simulink model "gm_uz_pmsm_model_6LUT_pd_vnl"  (R2023b)
settings: Solver=FixedStepAuto  StartTime=0.0  StopTime=0.05  RelTol=1e-3
PreLoadFcn:
  | uz_pmsm_model_init_parameter
PostLoadFcn:
  | % Import the data from Excel for a lookup table
  | FluxMapData = readtable('C:\Users\Philipp\ultrazohm\ultrazohm_sw\ip_cores\uz_pmsm_model\FluxMapData_2023-05-26_13-07-57.csv');
  | % Row indices for lookup table
  | d_current_in_d_axis = FluxMapData(8:27,1:end);
  | % Column indices for lookup table
  | q_current_in_d_axis = FluxMapData(29:48,1:end);
  | % Output values for lookup table
  | d_Flux_d_axis = FluxMapData(50:69,1:end);
undefined symbols (not defined in the file or in its folder): ad1, ad2, ad3, ad4, ad5, ad6, aq1, aq2, aq3, aq4, aq5, aq6, d_current_d_Flux, d_current_q_Flux, entkopplung_dynamic, entkopplung_linear, entkopplung_static, Fid1_Giq1, Fid2_Giq2, Flux_d, Flux_q, friction_coefficient, inertia, Ki_Bo_d, Ki_Bo_q, Kp_Bo_d, Kp_Bo_q, L_d, L_q, Ldq, parameter_nachfuerung, polepair, praediktion_entkopplung_nonlinear, psi_pm, q_current_d_Flux, q_current_q_Flux, R_1, simulate_mechanical, simulate_nonlinear_modell, simulate_open_loop, static_friction_torque, tau_sum, ts, ts_regler
libraries: hdlmdlgenlib x21, simulink x2, slpidlib x2
(part 3 of 4)

== system gm_uz_pmsm_model_6LUT_pd_vnl/uz_pmsm_model/Product110 ==
  In1 : Inport
  In2 : Inport  Port=2
  Product110 : Product  Inputs=**  OutDataTypeStr=single  SampleTime=1e-08
  Product110_pd1 : Delay  DelayLength=6
  Out1 : Outport
  wires:
  Product110_pd1/1 -> Out1/1
  Product110/1 -> Product110_pd1/1
  In2/1 -> Product110/2
  In1/1 -> Product110/1

== system gm_uz_pmsm_model_6LUT_pd_vnl/uz_pmsm_model/Product111 ==
  In1 : Inport
  In2 : Inport  Port=2
  Product111 : Product  Inputs=**  OutDataTypeStr=single  SampleTime=1e-08
  Product111_pd1 : Delay  DelayLength=6
  Out1 : Outport
  wires:
  Product111_pd1/1 -> Out1/1
  Product111/1 -> Product111_pd1/1
  In2/1 -> Product111/2
  In1/1 -> Product111/1

== system gm_uz_pmsm_model_6LUT_pd_vnl/uz_pmsm_model/Product12 ==
  In1 : Inport
  In2 : Inport  Port=2
  Product12 : Product  Inputs=**  OutDataTypeStr=single  SampleTime=1e-08
  Product12_pd1 : Delay  DelayLength=6
  Out1 : Outport
  wires:
  Product12_pd1/1 -> Out1/1
  Product12/1 -> Product12_pd1/1
  In2/1 -> Product12/2
  In1/1 -> Product12/1

== system gm_uz_pmsm_model_6LUT_pd_vnl/uz_pmsm_model/Product121 ==
  In1 : Inport
  In2 : Inport  Port=2
  Product121 : Product  Inputs=**  OutDataTypeStr=single  SampleTime=1e-08
  Product121_pd1 : Delay  DelayLength=6
  Out1 : Outport
  wires:
  Product121_pd1/1 -> Out1/1
  Product121/1 -> Product121_pd1/1
  In2/1 -> Product121/2
  In1/1 -> Product121/1

== system gm_uz_pmsm_model_6LUT_pd_vnl/uz_pmsm_model/Product122 ==
  In1 : Inport
  In2 : Inport  Port=2
  Product122 : Product  Inputs=**  OutDataTypeStr=single  SampleTime=1e-08
  Product122_pd1 : Delay  DelayLength=6
  Out1 : Outport
  wires:
  Product122_pd1/1 -> Out1/1
  Product122/1 -> Product122_pd1/1
  In2/1 -> Product122/2
  In1/1 -> Product122/1

== system gm_uz_pmsm_model_6LUT_pd_vnl/uz_pmsm_model/Product13 ==
  In1 : Inport
  In2 : Inport  Port=2
  Product13 : Product  Inputs=**  OutDataTypeStr=single  SampleTime=1e-08
  Product13_pd1 : Delay  DelayLength=6
  Out1 : Outport
  wires:
  Product13_pd1/1 -> Out1/1
  Product13/1 -> Product13_pd1/1
  In2/1 -> Product13/2
  In1/1 -> Product13/1

== system gm_uz_pmsm_model_6LUT_pd_vnl/uz_pmsm_model/Product131 ==
  In1 : Inport
  In2 : Inport  Port=2
  Product131 : Product  Inputs=**  OutDataTypeStr=single  SampleTime=1e-08
  Product131_pd1 : Delay  DelayLength=6
  Out1 : Outport
  wires:
  Product131_pd1/1 -> Out1/1
  Product131/1 -> Product131_pd1/1
  In2/1 -> Product131/2
  In1/1 -> Product131/1

== system gm_uz_pmsm_model_6LUT_pd_vnl/uz_pmsm_model/Product14 ==
  In1 : Inport
  In2 : Inport  Port=2
  Product14 : Product  Inputs=**  OutDataTypeStr=single  SampleTime=1e-08
  Product14_pd1 : Delay  DelayLength=6
  Out1 : Outport
  wires:
  Product14_pd1/1 -> Out1/1
  Product14/1 -> Product14_pd1/1
  In2/1 -> Product14/2
  In1/1 -> Product14/1

== system gm_uz_pmsm_model_6LUT_pd_vnl/uz_pmsm_model/Product141 ==
  In1 : Inport
  In2 : Inport  Port=2
  Product141 : Product  Inputs=**  OutDataTypeStr=single  SampleTime=1e-08
  Product141_pd1 : Delay  DelayLength=6
  Out1 : Outport
  wires:
  Product141_pd1/1 -> Out1/1
  Product141/1 -> Product141_pd1/1
  In2/1 -> Product141/2
  In1/1 -> Product141/1

== system gm_uz_pmsm_model_6LUT_pd_vnl/uz_pmsm_model/Product142 ==
  In1 : Inport
  In2 : Inport  Port=2
  Product142 : Product  Inputs=**  OutDataTypeStr=single  SampleTime=1e-08
  Product142_pd1 : Delay  DelayLength=6
  Out1 : Outport
  wires:
  Product142_pd1/1 -> Out1/1
  Product142/1 -> Product142_pd1/1
  In2/1 -> Product142/2
  In1/1 -> Product142/1

== system gm_uz_pmsm_model_6LUT_pd_vnl/uz_pmsm_model/Product15 ==
  In1 : Inport
  In2 : Inport  Port=2
  Product15 : Product  Inputs=**  OutDataTypeStr=single  SampleTime=1e-08
  Product15_pd1 : Delay  DelayLength=6
  Out1 : Outport
  wires:
  Product15_pd1/1 -> Out1/1
  Product15/1 -> Product15_pd1/1
  In2/1 -> Product15/2
  In1/1 -> Product15/1

== system gm_uz_pmsm_model_6LUT_pd_vnl/uz_pmsm_model/Product151 ==
  In1 : Inport
  In2 : Inport  Port=2
  Product151 : Product  Inputs=**  OutDataTypeStr=single  SampleTime=1e-08
  Product151_pd1 : Delay  DelayLength=6
  Out1 : Outport
  wires:
  Product151_pd1/1 -> Out1/1
  Product151/1 -> Product151_pd1/1
  In2/1 -> Product151/2
  In1/1 -> Product151/1

== system gm_uz_pmsm_model_6LUT_pd_vnl/uz_pmsm_model/Product16 ==
  In1 : Inport
  In2 : Inport  Port=2
  Product16 : Product  Inputs=**  OutDataTypeStr=single  SampleTime=1e-08
  Product16_pd1 : Delay  DelayLength=6
  Out1 : Outport
  wires:
  Product16_pd1/1 -> Out1/1
  Product16/1 -> Product16_pd1/1
  In2/1 -> Product16/2
  In1/1 -> Product16/1

== system gm_uz_pmsm_model_6LUT_pd_vnl/uz_pmsm_model/Product17 ==
  In1 : Inport
  In2 : Inport  Port=2
  Product17 : Product  Inputs=**  OutDataTypeStr=single  SampleTime=1e-08
  Product17_pd1 : Delay  DelayLength=6
  Out1 : Outport
  wires:
  Product17_pd1/1 -> Out1/1
  Product17/1 -> Product17_pd1/1
  In2/1 -> Product17/2
  In1/1 -> Product17/1

== system gm_uz_pmsm_model_6LUT_pd_vnl/uz_pmsm_model/Product18 ==
  In1 : Inport
  In2 : Inport  Port=2
  Product18 : Product  Inputs=**  OutDataTypeStr=single  SampleTime=1e-08
  Product18_pd1 : Delay  DelayLength=6
  Out1 : Outport
  wires:
  Product18_pd1/1 -> Out1/1
  Product18/1 -> Product18_pd1/1
  In2/1 -> Product18/2
  In1/1 -> Product18/1

== system gm_uz_pmsm_model_6LUT_pd_vnl/uz_pmsm_model/Product19 ==
  In1 : Inport
  In2 : Inport  Port=2
  Product19 : Product  Inputs=**  OutDataTypeStr=single  SampleTime=1e-08
  Product19_pd1 : Delay  DelayLength=6
  Out1 : Outport
  wires:
  Product19_pd1/1 -> Out1/1
  Product19/1 -> Product19_pd1/1
  In2/1 -> Product19/2
  In1/1 -> Product19/1

== system gm_uz_pmsm_model_6LUT_pd_vnl/uz_pmsm_model/Product2 ==
  In1 : Inport
  In2 : Inport  Port=2
  Product2 : Product  Inputs=**  OutDataTypeStr=single  SampleTime=1e-08
  Product2_pd1 : Delay  DelayLength=6
  Out1 : Outport
  wires:
  Product2_pd1/1 -> Out1/1
  Product2/1 -> Product2_pd1/1
  In2/1 -> Product2/2
  In1/1 -> Product2/1

== system gm_uz_pmsm_model_6LUT_pd_vnl/uz_pmsm_model/Product20 ==
  In1 : Inport
  In2 : Inport  Port=2
  Product20 : Product  Inputs=**  OutDataTypeStr=single  SampleTime=1e-08
  Product20_pd1 : Delay  DelayLength=6
  Out1 : Outport
  wires:
  Product20_pd1/1 -> Out1/1
  Product20/1 -> Product20_pd1/1
  In2/1 -> Product20/2
  In1/1 -> Product20/1

== system gm_uz_pmsm_model_6LUT_pd_vnl/uz_pmsm_model/Product201 ==
  In1 : Inport
  In2 : Inport  Port=2
  Product201 : Product  Inputs=**  OutDataTypeStr=single  SampleTime=1e-08
  Product201_pd1 : Delay  DelayLength=6
  Out1 : Outport
  wires:
  Product201_pd1/1 -> Out1/1
  Product201/1 -> Product201_pd1/1
  In2/1 -> Product201/2
  In1/1 -> Product201/1

== system gm_uz_pmsm_model_6LUT_pd_vnl/uz_pmsm_model/Product202 ==
  In1 : Inport
  In2 : Inport  Port=2
  Product202 : Product  Inputs=**  OutDataTypeStr=single  SampleTime=1e-08
  Product202_pd1 : Delay  DelayLength=6
  Out1 : Outport
  wires:
  Product202_pd1/1 -> Out1/1
  Product202/1 -> Product202_pd1/1
  In2/1 -> Product202/2
  In1/1 -> Product202/1

== system gm_uz_pmsm_model_6LUT_pd_vnl/uz_pmsm_model/Product203 ==
  In1 : Inport
  In2 : Inport  Port=2
  Product203 : Product  Inputs=**  OutDataTypeStr=single  SampleTime=1e-08
  Product203_pd1 : Delay  DelayLength=6
  Out1 : Outport
  wires:
  Product203_pd1/1 -> Out1/1
  Product203/1 -> Product203_pd1/1
  In2/1 -> Product203/2
  In1/1 -> Product203/1

== system gm_uz_pmsm_model_6LUT_pd_vnl/uz_pmsm_model/Product204 ==
  In1 : Inport
  In2 : Inport  Port=2
  Product204 : Product  Inputs=**  OutDataTypeStr=single  SampleTime=1e-08
  Product204_pd1 : Delay  DelayLength=6
  Out1 : Outport
  wires:
  Product204_pd1/1 -> Out1/1
  Product204/1 -> Product204_pd1/1
  In2/1 -> Product204/2
  In1/1 -> Product204/1

== system gm_uz_pmsm_model_6LUT_pd_vnl/uz_pmsm_model/Product205 ==
  In1 : Inport
  In2 : Inport  Port=2
  Product205 : Product  Inputs=**  OutDataTypeStr=single  SampleTime=1e-08
  Product205_pd1 : Delay  DelayLength=6
  Out1 : Outport
  wires:
  Product205_pd1/1 -> Out1/1
  Product205/1 -> Product205_pd1/1
  In2/1 -> Product205/2
  In1/1 -> Product205/1

== system gm_uz_pmsm_model_6LUT_pd_vnl/uz_pmsm_model/Product206 ==
  In1 : Inport
  In2 : Inport  Port=2
  Product206 : Product  Inputs=**  OutDataTypeStr=single  SampleTime=1e-08
  Product206_pd1 : Delay  DelayLength=6
  Out1 : Outport
  wires:
  Product206_pd1/1 -> Out1/1
  Product206/1 -> Product206_pd1/1
  In2/1 -> Product206/2
  In1/1 -> Product206/1

== system gm_uz_pmsm_model_6LUT_pd_vnl/uz_pmsm_model/Product207 ==
  In1 : Inport
  In2 : Inport  Port=2
  Product207 : Product  Inputs=**  OutDataTypeStr=single  SampleTime=1e-08
  Product207_pd1 : Delay  DelayLength=6
  Out1 : Outport
  wires:
  Product207_pd1/1 -> Out1/1
  Product207/1 -> Product207_pd1/1
  In2/1 -> Product207/2
  In1/1 -> Product207/1

== system gm_uz_pmsm_model_6LUT_pd_vnl/uz_pmsm_model/Product21 ==
  In1 : Inport
  In2 : Inport  Port=2
  Product21 : Product  Inputs=**  OutDataTypeStr=single  SampleTime=1e-08
  Product21_pd1 : Delay  DelayLength=6
  Out1 : Outport
  wires:
  Product21_pd1/1 -> Out1/1
  Product21/1 -> Product21_pd1/1
  In2/1 -> Product21/2
  In1/1 -> Product21/1

== system gm_uz_pmsm_model_6LUT_pd_vnl/uz_pmsm_model/Product22 ==
  In1 : Inport
  In2 : Inport  Port=2
  Product22 : Product  Inputs=**  OutDataTypeStr=single  SampleTime=1e-08
  Product22_pd1 : Delay  DelayLength=6
  Out1 : Outport
  wires:
  Product22_pd1/1 -> Out1/1
  Product22/1 -> Product22_pd1/1
  In2/1 -> Product22/2
  In1/1 -> Product22/1

== system gm_uz_pmsm_model_6LUT_pd_vnl/uz_pmsm_model/Product23 ==
  In1 : Inport
  In2 : Inport  Port=2
  Product23 : Product  Inputs=**  OutDataTypeStr=single  SampleTime=1e-08
  Product23_pd1 : Delay  DelayLength=6
  Out1 : Outport
  wires:
  Product23_pd1/1 -> Out1/1
  Product23/1 -> Product23_pd1/1
  In2/1 -> Product23/2
  In1/1 -> Product23/1

== system gm_uz_pmsm_model_6LUT_pd_vnl/uz_pmsm_model/Product24 ==
  In1 : Inport
  In2 : Inport  Port=2
  Product24 : Product  Inputs=**  OutDataTypeStr=single  SampleTime=1e-08
  Product24_pd1 : Delay  DelayLength=6
  Out1 : Outport
  wires:
  Product24_pd1/1 -> Out1/1
  Product24/1 -> Product24_pd1/1
  In2/1 -> Product24/2
  In1/1 -> Product24/1

== system gm_uz_pmsm_model_6LUT_pd_vnl/uz_pmsm_model/Product25 ==
  In1 : Inport
  In2 : Inport  Port=2
  Product25 : Product  Inputs=**  OutDataTypeStr=single  SampleTime=1e-08
  Product25_pd1 : Delay  DelayLength=6
  Out1 : Outport
  wires:
  Product25_pd1/1 -> Out1/1
  Product25/1 -> Product25_pd1/1
  In2/1 -> Product25/2
  In1/1 -> Product25/1

== system gm_uz_pmsm_model_6LUT_pd_vnl/uz_pmsm_model/Product3 ==
  In1 : Inport
  In2 : Inport  Port=2
  Product3 : Product  Inputs=**  OutDataTypeStr=single  SampleTime=1e-08
  Product3_pd1 : Delay  DelayLength=6
  Out1 : Outport
  wires:
  Product3_pd1/1 -> Out1/1
  Product3/1 -> Product3_pd1/1
  In2/1 -> Product3/2
  In1/1 -> Product3/1

== system gm_uz_pmsm_model_6LUT_pd_vnl/uz_pmsm_model/Product31 ==
  In1 : Inport
  In2 : Inport  Port=2
  Product31 : Product  Inputs=**  OutDataTypeStr=single  SampleTime=1e-08
  Product31_pd1 : Delay  DelayLength=6
  Out1 : Outport
  wires:
  Product31_pd1/1 -> Out1/1
  Product31/1 -> Product31_pd1/1
  In2/1 -> Product31/2
  In1/1 -> Product31/1

== system gm_uz_pmsm_model_6LUT_pd_vnl/uz_pmsm_model/Product32 ==
  In1 : Inport
  In2 : Inport  Port=2
  Product32 : Product  Inputs=**  OutDataTypeStr=single  SampleTime=1e-08
  Product32_pd1 : Delay  DelayLength=6
  Out1 : Outport
  wires:
  Product32_pd1/1 -> Out1/1
  Product32/1 -> Product32_pd1/1
  In2/1 -> Product32/2
  In1/1 -> Product32/1

== system gm_uz_pmsm_model_6LUT_pd_vnl/uz_pmsm_model/Product33 ==
  In1 : Inport
  In2 : Inport  Port=2
  Product33 : Product  Inputs=**  OutDataTypeStr=single  SampleTime=1e-08
  Product33_pd1 : Delay  DelayLength=6
  Out1 : Outport
  wires:
  Product33_pd1/1 -> Out1/1
  Product33/1 -> Product33_pd1/1
  In2/1 -> Product33/2
  In1/1 -> Product33/1

== system gm_uz_pmsm_model_6LUT_pd_vnl/uz_pmsm_model/Product34 ==
  In1 : Inport
  In2 : Inport  Port=2
  Product34 : Product  Inputs=**  OutDataTypeStr=single  SampleTime=1e-08
  Product34_pd1 : Delay  DelayLength=6
  Out1 : Outport
  wires:
  Product34_pd1/1 -> Out1/1
  Product34/1 -> Product34_pd1/1
  In2/1 -> Product34/2
  In1/1 -> Product34/1

== system gm_uz_pmsm_model_6LUT_pd_vnl/uz_pmsm_model/Product35 ==
  In1 : Inport
  In2 : Inport  Port=2
  Product35 : Product  Inputs=**  OutDataTypeStr=single  SampleTime=1e-08
  Product35_pd1 : Delay  DelayLength=6
  Out1 : Outport
  wires:
  Product35_pd1/1 -> Out1/1
  Product35/1 -> Product35_pd1/1
  In2/1 -> Product35/2
  In1/1 -> Product35/1

== system gm_uz_pmsm_model_6LUT_pd_vnl/uz_pmsm_model/Product4 ==
  In1 : Inport
  In2 : Inport  Port=2
  Product4 : Product  Inputs=**  OutDataTypeStr=single  SampleTime=1e-08
  Product4_pd1 : Delay  DelayLength=6
  Out1 : Outport
  wires:
  Product4_pd1/1 -> Out1/1
  Product4/1 -> Product4_pd1/1
  In2/1 -> Product4/2
  In1/1 -> Product4/1

== system gm_uz_pmsm_model_6LUT_pd_vnl/uz_pmsm_model/Product41 ==
  In1 : Inport
  In2 : Inport  Port=2
  Product41 : Product  Inputs=**  OutDataTypeStr=single  SampleTime=1e-08
  Product41_pd1 : Delay  DelayLength=6
  Out1 : Outport
  wires:
  Product41_pd1/1 -> Out1/1
  Product41/1 -> Product41_pd1/1
  In2/1 -> Product41/2
  In1/1 -> Product41/1

== system gm_uz_pmsm_model_6LUT_pd_vnl/uz_pmsm_model/Product42 ==
  In1 : Inport
  In2 : Inport  Port=2
  Product42 : Product  Inputs=**  OutDataTypeStr=single  SampleTime=1e-08
  Product42_pd1 : Delay  DelayLength=6
  Out1 : Outport
  wires:
  Product42_pd1/1 -> Out1/1
  Product42/1 -> Product42_pd1/1
  In2/1 -> Product42/2
  In1/1 -> Product42/1

== system gm_uz_pmsm_model_6LUT_pd_vnl/uz_pmsm_model/Product43 ==
  In1 : Inport
  In2 : Inport  Port=2
  Product43 : Product  Inputs=**  OutDataTypeStr=single  SampleTime=1e-08
  Product43_pd1 : Delay  DelayLength=6
  Out1 : Outport
  wires:
  Product43_pd1/1 -> Out1/1
  Product43/1 -> Product43_pd1/1
  In2/1 -> Product43/2
  In1/1 -> Product43/1

== system gm_uz_pmsm_model_6LUT_pd_vnl/uz_pmsm_model/Product5 ==
  In1 : Inport
  In2 : Inport  Port=2
  Product5 : Product  Inputs=**  OutDataTypeStr=single  SampleTime=1e-08
  Product5_pd1 : Delay  DelayLength=6
  Out1 : Outport
  wires:
  Product5_pd1/1 -> Out1/1
  Product5/1 -> Product5_pd1/1
  In2/1 -> Product5/2
  In1/1 -> Product5/1

== system gm_uz_pmsm_model_6LUT_pd_vnl/uz_pmsm_model/Product51 ==
  In1 : Inport
  In2 : Inport  Port=2
  Product51 : Product  Inputs=**  OutDataTypeStr=single  SampleTime=1e-08
  Product51_pd1 : Delay  DelayLength=6
  Out1 : Outport
  wires:
  Product51_pd1/1 -> Out1/1
  Product51/1 -> Product51_pd1/1
  In2/1 -> Product51/2
  In1/1 -> Product51/1

== system gm_uz_pmsm_model_6LUT_pd_vnl/uz_pmsm_model/Product52 ==
  In1 : Inport
  In2 : Inport  Port=2
  Product52 : Product  Inputs=**  OutDataTypeStr=single  SampleTime=1e-08
  Product52_pd1 : Delay  DelayLength=6
  Out1 : Outport
  wires:
  Product52_pd1/1 -> Out1/1
  Product52/1 -> Product52_pd1/1
  In2/1 -> Product52/2
  In1/1 -> Product52/1

== system gm_uz_pmsm_model_6LUT_pd_vnl/uz_pmsm_model/Product6 ==
  In1 : Inport
  In2 : Inport  Port=2
  Product6 : Product  Inputs=**  OutDataTypeStr=single  SampleTime=1e-08
  Product6_pd1 : Delay  DelayLength=6
  Out1 : Outport
  wires:
  Product6_pd1/1 -> Out1/1
  Product6/1 -> Product6_pd1/1
  In2/1 -> Product6/2
  In1/1 -> Product6/1

== system gm_uz_pmsm_model_6LUT_pd_vnl/uz_pmsm_model/Product61 ==
  In1 : Inport
  In2 : Inport  Port=2
  Product61 : Product  Inputs=**  OutDataTypeStr=single  SampleTime=1e-08
  Product61_pd1 : Delay  DelayLength=6
  Out1 : Outport
  wires:
  Product61_pd1/1 -> Out1/1
  Product61/1 -> Product61_pd1/1
  In2/1 -> Product61/2
  In1/1 -> Product61/1

== system gm_uz_pmsm_model_6LUT_pd_vnl/uz_pmsm_model/Product7 ==
  In1 : Inport
  In2 : Inport  Port=2
  Product7 : Product  Inputs=**  OutDataTypeStr=single  SampleTime=1e-08
  Product7_pd1 : Delay  DelayLength=6
  Out1 : Outport
  wires:
  Product7_pd1/1 -> Out1/1
  Product7/1 -> Product7_pd1/1
  In2/1 -> Product7/2
  In1/1 -> Product7/1

== system gm_uz_pmsm_model_6LUT_pd_vnl/uz_pmsm_model/Product71 ==
  In1 : Inport
  In2 : Inport  Port=2
  Product71 : Product  Inputs=**  OutDataTypeStr=single  SampleTime=1e-08
  Product71_pd1 : Delay  DelayLength=6
  Out1 : Outport
  wires:
  Product71_pd1/1 -> Out1/1
  Product71/1 -> Product71_pd1/1
  In2/1 -> Product71/2
  In1/1 -> Product71/1

== system gm_uz_pmsm_model_6LUT_pd_vnl/uz_pmsm_model/Product8 ==
  In1 : Inport
  In2 : Inport  Port=2
  Product8 : Product  Inputs=**  OutDataTypeStr=single  SampleTime=1e-08
  Product8_pd1 : Delay  DelayLength=6
  Out1 : Outport
  wires:
  Product8_pd1/1 -> Out1/1
  Product8/1 -> Product8_pd1/1
  In2/1 -> Product8/2
  In1/1 -> Product8/1

== system gm_uz_pmsm_model_6LUT_pd_vnl/uz_pmsm_model/Product9 ==
  In1 : Inport
  In2 : Inport  Port=2
  Product9 : Product  Inputs=**  OutDataTypeStr=single  SampleTime=1e-08
  Product9_pd1 : Delay  DelayLength=6
  Out1 : Outport
  wires:
  Product9_pd1/1 -> Out1/1
  Product9/1 -> Product9_pd1/1
  In2/1 -> Product9/2
  In1/1 -> Product9/1

== system gm_uz_pmsm_model_6LUT_pd_vnl/uz_pmsm_model/Product91 ==
  In1 : Inport
  In2 : Inport  Port=2
  Product91 : Product  Inputs=**  OutDataTypeStr=single  SampleTime=1e-08
  Product91_pd1 : Delay  DelayLength=6
  Out1 : Outport
  wires:
  Product91_pd1/1 -> Out1/1
  Product91/1 -> Product91_pd1/1
  In2/1 -> Product91/2
  In1/1 -> Product91/1

== system gm_uz_pmsm_model_6LUT_pd_vnl/uz_pmsm_model/Product92 ==
  In1 : Inport
  In2 : Inport  Port=2
  Product92 : Product  Inputs=**  OutDataTypeStr=single  SampleTime=1e-08
  Product92_pd1 : Delay  DelayLength=6
  Out1 : Outport
  wires:
  Product92_pd1/1 -> Out1/1
  Product92/1 -> Product92_pd1/1
  In2/1 -> Product92/2
  In1/1 -> Product92/1

== system gm_uz_pmsm_model_6LUT_pd_vnl/uz_pmsm_model/Reciprocal1_recip ==
  In1 : Inport
  Reciprocal1_recip : Math  Operator=reciprocal  SampleTime=1e-08
  Reciprocal1_recip_pd1 : Delay  DelayLength=16
  Out1 : Outport
  wires:
  Reciprocal1_recip_pd1/1 -> Out1/1
  Reciprocal1_recip/1 -> Reciprocal1_recip_pd1/1
  In1/1 -> Reciprocal1_recip/1

== system gm_uz_pmsm_model_6LUT_pd_vnl/uz_pmsm_model/Reciprocal1_recip1 ==
  In1 : Inport
  Reciprocal1_recip1 : Math  Operator=reciprocal  SampleTime=1e-08
  Reciprocal1_recip1_pd1 : Delay  DelayLength=16
  Out1 : Outport
  wires:
  Reciprocal1_recip1_pd1/1 -> Out1/1
  Reciprocal1_recip1/1 -> Reciprocal1_recip1_pd1/1
  In1/1 -> Reciprocal1_recip1/1

== system gm_uz_pmsm_model_6LUT_pd_vnl/uz_pmsm_model/Reciprocal_recip ==
  In1 : Inport
  Reciprocal_recip : Math  Operator=reciprocal  SampleTime=1e-08
  Reciprocal_recip_pd1 : Delay  DelayLength=16
  Out1 : Outport
  wires:
  Reciprocal_recip_pd1/1 -> Out1/1
  Reciprocal_recip/1 -> Reciprocal_recip_pd1/1
  In1/1 -> Reciprocal_recip/1

== system gm_uz_pmsm_model_6LUT_pd_vnl/uz_pmsm_model/Reciprocal_recip1 ==
  In1 : Inport
  Reciprocal_recip1 : Math  Operator=reciprocal  SampleTime=1e-08
  Reciprocal_recip1_pd1 : Delay  DelayLength=16
  Out1 : Outport
  wires:
  Reciprocal_recip1_pd1/1 -> Out1/1
  Reciprocal_recip1/1 -> Reciprocal_recip1_pd1/1
  In1/1 -> Reciprocal_recip1/1

== system gm_uz_pmsm_model_6LUT_pd_vnl/uz_pmsm_model/Sign1 ==
  In1 : Inport
  Sign1 : Signum  SampleTime=1e-08
  Out1 : Outport
  wires:
  Sign1/1 -> Out1/1
  In1/1 -> Sign1/1

== system gm_uz_pmsm_model_6LUT_pd_vnl/uz_pmsm_model/Sum ==
  In1 : Inport
  In2 : Inport  Port=2
  Sum : Sum  OutDataTypeStr=single  SampleTime=1e-08
  Sum_pd1 : Delay  DelayLength=6
  Out1 : Outport
  wires:
  Sum_pd1/1 -> Out1/1
  Sum/1 -> Sum_pd1/1
  In2/1 -> Sum/2
  In1/1 -> Sum/1

== system gm_uz_pmsm_model_6LUT_pd_vnl/uz_pmsm_model/Sum1 ==
  In1 : Inport
  In2 : Inport  Port=2
  Sum1 : Sum  Inputs=+-  OutDataTypeStr=single  SampleTime=1e-08
  Sum1_pd1 : Delay  DelayLength=6
  Out1 : Outport
  wires:
  Sum1_pd1/1 -> Out1/1
  Sum1/1 -> Sum1_pd1/1
  In2/1 -> Sum1/2
  In1/1 -> Sum1/1

== system gm_uz_pmsm_model_6LUT_pd_vnl/uz_pmsm_model/Sum10 ==
  In1 : Inport
  In2 : Inport  Port=2
  Sum10 : Sum  Inputs=+-  OutDataTypeStr=single  SampleTime=1e-08
  Sum10_pd1 : Delay  DelayLength=6
  Out1 : Outport
  wires:
  Sum10_pd1/1 -> Out1/1
  Sum10/1 -> Sum10_pd1/1
  In2/1 -> Sum10/2
  In1/1 -> Sum10/1

== system gm_uz_pmsm_model_6LUT_pd_vnl/uz_pmsm_model/Sum101 ==
  In1 : Inport
  In2 : Inport  Port=2
  Sum101 : Sum  Inputs=+-  OutDataTypeStr=single  SampleTime=1e-08
  Sum101_pd1 : Delay  DelayLength=6
  Out1 : Outport
  wires:
  Sum101_pd1/1 -> Out1/1
  Sum101/1 -> Sum101_pd1/1
  In2/1 -> Sum101/2
  In1/1 -> Sum101/1

== system gm_uz_pmsm_model_6LUT_pd_vnl/uz_pmsm_model/Sum11 ==
  In1 : Inport
  In2 : Inport  Port=2
  Sum11 : Sum  Inputs=+-  OutDataTypeStr=single  SampleTime=1e-08
  Sum11_pd1 : Delay  DelayLength=6
  Out1 : Outport
  wires:
  Sum11_pd1/1 -> Out1/1
  Sum11/1 -> Sum11_pd1/1
  In2/1 -> Sum11/2
  In1/1 -> Sum11/1

== system gm_uz_pmsm_model_6LUT_pd_vnl/uz_pmsm_model/Sum12 ==
  In1 : Inport
  In2 : Inport  Port=2
  Sum12 : Sum  OutDataTypeStr=single  SampleTime=1e-08
  Sum12_pd1 : Delay  DelayLength=6
  Out1 : Outport
  wires:
  Sum12_pd1/1 -> Out1/1
  Sum12/1 -> Sum12_pd1/1
  In2/1 -> Sum12/2
  In1/1 -> Sum12/1

== system gm_uz_pmsm_model_6LUT_pd_vnl/uz_pmsm_model/Sum13 ==
  In1 : Inport
  In2 : Inport  Port=2
  Sum13 : Sum  OutDataTypeStr=single  SampleTime=1e-08
  Sum13_pd1 : Delay  DelayLength=6
  Out1 : Outport
  wires:
  Sum13_pd1/1 -> Out1/1
  Sum13/1 -> Sum13_pd1/1
  In2/1 -> Sum13/2
  In1/1 -> Sum13/1

== system gm_uz_pmsm_model_6LUT_pd_vnl/uz_pmsm_model/Sum14 ==
  In1 : Inport
  In2 : Inport  Port=2
  Sum14 : Sum  Inputs=+-  OutDataTypeStr=single  SampleTime=1e-08
  Sum14_pd1 : Delay  DelayLength=6
  Out1 : Outport
  wires:
  Sum14_pd1/1 -> Out1/1
  Sum14/1 -> Sum14_pd1/1
  In2/1 -> Sum14/2
  In1/1 -> Sum14/1

== system gm_uz_pmsm_model_6LUT_pd_vnl/uz_pmsm_model/Sum2 ==
  In1 : Inport
  In2 : Inport  Port=2
  Sum2 : Sum  Inputs=+-  OutDataTypeStr=single  SampleTime=1e-08
  Sum2_pd1 : Delay  DelayLength=6
  Out1 : Outport
  wires:
  Sum2_pd1/1 -> Out1/1
  Sum2/1 -> Sum2_pd1/1
  In2/1 -> Sum2/2
  In1/1 -> Sum2/1

== system gm_uz_pmsm_model_6LUT_pd_vnl/uz_pmsm_model/Sum21 ==
  In1 : Inport
  In2 : Inport  Port=2
  Sum21 : Sum  Inputs=+-  OutDataTypeStr=single  SampleTime=1e-08
  Sum21_pd1 : Delay  DelayLength=6
  Out1 : Outport
  wires:
  Sum21_pd1/1 -> Out1/1
  Sum21/1 -> Sum21_pd1/1
  In2/1 -> Sum21/2
  In1/1 -> Sum21/1

== system gm_uz_pmsm_model_6LUT_pd_vnl/uz_pmsm_model/Sum22 ==
  In1 : Inport
  In2 : Inport  Port=2
  Sum22 : Sum  Inputs=+-  OutDataTypeStr=single  SampleTime=1e-08
  Sum22_pd1 : Delay  DelayLength=6
  Out1 : Outport
  wires:
  Sum22_pd1/1 -> Out1/1
  Sum22/1 -> Sum22_pd1/1
  In2/1 -> Sum22/2
  In1/1 -> Sum22/1

== system gm_uz_pmsm_model_6LUT_pd_vnl/uz_pmsm_model/Sum23 ==
  In1 : Inport
  In2 : Inport  Port=2
  Sum23 : Sum  Inputs=+-  OutDataTypeStr=single  SampleTime=1e-08
  Sum23_pd1 : Delay  DelayLength=6
  Out1 : Outport
  wires:
  Sum23_pd1/1 -> Out1/1
  Sum23/1 -> Sum23_pd1/1
  In2/1 -> Sum23/2
  In1/1 -> Sum23/1

== system gm_uz_pmsm_model_6LUT_pd_vnl/uz_pmsm_model/Sum3 ==
  In1 : Inport
  In2 : Inport  Port=2
  Sum3 : Sum  Inputs=+-  OutDataTypeStr=single  SampleTime=1e-08
  Sum3_pd1 : Delay  DelayLength=6
  Out1 : Outport
  wires:
  Sum3_pd1/1 -> Out1/1
  Sum3/1 -> Sum3_pd1/1
  In2/1 -> Sum3/2
  In1/1 -> Sum3/1

== system gm_uz_pmsm_model_6LUT_pd_vnl/uz_pmsm_model/Sum31 ==
  In1 : Inport
  In2 : Inport  Port=2
  Sum31 : Sum  Inputs=+-  OutDataTypeStr=single  SampleTime=1e-08
  Sum31_pd1 : Delay  DelayLength=6
  Out1 : Outport
  wires:
  Sum31_pd1/1 -> Out1/1
  Sum31/1 -> Sum31_pd1/1
  In2/1 -> Sum31/2
  In1/1 -> Sum31/1

== system gm_uz_pmsm_model_6LUT_pd_vnl/uz_pmsm_model/Sum32 ==
  In1 : Inport
  In2 : Inport  Port=2
  Sum32 : Sum  OutDataTypeStr=single  SampleTime=1e-08
  Sum32_pd1 : Delay  DelayLength=6
  Out1 : Outport
  wires:
  Sum32_pd1/1 -> Out1/1
  Sum32/1 -> Sum32_pd1/1
  In2/1 -> Sum32/2
  In1/1 -> Sum32/1

== system gm_uz_pmsm_model_6LUT_pd_vnl/uz_pmsm_model/Sum33 ==
  In1 : Inport
  In2 : Inport  Port=2
  Sum33 : Sum  Inputs=+-  OutDataTypeStr=single  SampleTime=1e-08
  Sum33_pd1 : Delay  DelayLength=6
  Out1 : Outport
  wires:
  Sum33_pd1/1 -> Out1/1
  Sum33/1 -> Sum33_pd1/1
  In2/1 -> Sum33/2
  In1/1 -> Sum33/1

== system gm_uz_pmsm_model_6LUT_pd_vnl/uz_pmsm_model/Sum3_stage2 ==
  In1 : Inport
  In2 : Inport  Port=2
  Sum3_stage2 : Sum  OutDataTypeStr=single  SampleTime=1e-08
  Sum3_stage2_pd1 : Delay  DelayLength=6
  Out1 : Outport
  wires:
  Sum3_stage2_pd1/1 -> Out1/1
  Sum3_stage2/1 -> Sum3_stage2_pd1/1
  In2/1 -> Sum3_stage2/2
  In1/1 -> Sum3_stage2/1

== system gm_uz_pmsm_model_6LUT_pd_vnl/uz_pmsm_model/Sum3_stage21 ==
  In1 : Inport
  In2 : Inport  Port=2
  Sum3_stage21 : Sum  Inputs=+-  OutDataTypeStr=single  SampleTime=1e-08
  Sum3_stage21_pd1 : Delay  DelayLength=6
  Out1 : Outport
  wires:
  Sum3_stage21_pd1/1 -> Out1/1
  Sum3_stage21/1 -> Sum3_stage21_pd1/1
  In2/1 -> Sum3_stage21/2
  In1/1 -> Sum3_stage21/1

== system gm_uz_pmsm_model_6LUT_pd_vnl/uz_pmsm_model/Sum3_stage3 ==
  In1 : Inport
  In2 : Inport  Port=2
  Sum3_stage3 : Sum  Inputs=+-  OutDataTypeStr=single  SampleTime=1e-08
  Sum3_stage3_pd1 : Delay  DelayLength=6
  Out1 : Outport
  wires:
  Sum3_stage3_pd1/1 -> Out1/1
  Sum3_stage3/1 -> Sum3_stage3_pd1/1
  In2/1 -> Sum3_stage3/2
  In1/1 -> Sum3_stage3/1

== system gm_uz_pmsm_model_6LUT_pd_vnl/uz_pmsm_model/Sum3_stage31 ==
  In1 : Inport
  In2 : Inport  Port=2
  Sum3_stage31 : Sum  Inputs=+-  OutDataTypeStr=single  SampleTime=1e-08
  Sum3_stage31_pd1 : Delay  DelayLength=6
  Out1 : Outport
  wires:
  Sum3_stage31_pd1/1 -> Out1/1
  Sum3_stage31/1 -> Sum3_stage31_pd1/1
  In2/1 -> Sum3_stage31/2
  In1/1 -> Sum3_stage31/1

== system gm_uz_pmsm_model_6LUT_pd_vnl/uz_pmsm_model/Sum3_stage4 ==
  In1 : Inport
  In2 : Inport  Port=2
  Sum3_stage4 : Sum  OutDataTypeStr=single  SampleTime=1e-08
  Sum3_stage4_pd1 : Delay  DelayLength=6
  Out1 : Outport
  wires:
  Sum3_stage4_pd1/1 -> Out1/1
  Sum3_stage4/1 -> Sum3_stage4_pd1/1
  In2/1 -> Sum3_stage4/2
  In1/1 -> Sum3_stage4/1

== system gm_uz_pmsm_model_6LUT_pd_vnl/uz_pmsm_model/Sum4 ==
  In1 : Inport
  In2 : Inport  Port=2
  Sum4 : Sum  Inputs=+-  OutDataTypeStr=single  SampleTime=1e-08
  Sum4_pd1 : Delay  DelayLength=6
  Out1 : Outport
  wires:
  Sum4_pd1/1 -> Out1/1
  Sum4/1 -> Sum4_pd1/1
  In2/1 -> Sum4/2
  In1/1 -> Sum4/1

== system gm_uz_pmsm_model_6LUT_pd_vnl/uz_pmsm_model/Sum41 ==
  In1 : Inport
  In2 : Inport  Port=2
  Sum41 : Sum  OutDataTypeStr=single  SampleTime=1e-08
  Sum41_pd1 : Delay  DelayLength=6
  Out1 : Outport
  wires:
  Sum41_pd1/1 -> Out1/1
  Sum41/1 -> Sum41_pd1/1
  In2/1 -> Sum41/2
  In1/1 -> Sum41/1

== system gm_uz_pmsm_model_6LUT_pd_vnl/uz_pmsm_model/Sum42 ==
  In1 : Inport
  In2 : Inport  Port=2
  Sum42 : Sum  OutDataTypeStr=single  SampleTime=1e-08
  Sum42_pd1 : Delay  DelayLength=6
  Out1 : Outport
  wires:
  Sum42_pd1/1 -> Out1/1
  Sum42/1 -> Sum42_pd1/1
  In2/1 -> Sum42/2
  In1/1 -> Sum42/1

== system gm_uz_pmsm_model_6LUT_pd_vnl/uz_pmsm_model/Sum4_stage2 ==
  In1 : Inport
  In2 : Inport  Port=2
  Sum4_stage2 : Sum  Inputs=+-  OutDataTypeStr=single  SampleTime=1e-08
  Sum4_stage2_pd1 : Delay  DelayLength=6
  Out1 : Outport
  wires:
  Sum4_stage2_pd1/1 -> Out1/1
  Sum4_stage2/1 -> Sum4_stage2_pd1/1
  In2/1 -> Sum4_stage2/2
  In1/1 -> Sum4_stage2/1

== system gm_uz_pmsm_model_6LUT_pd_vnl/uz_pmsm_model/Sum4_stage3 ==
  In1 : Inport
  In2 : Inport  Port=2
  Sum4_stage3 : Sum  Inputs=+-  OutDataTypeStr=single  SampleTime=1e-08
  Sum4_stage3_pd1 : Delay  DelayLength=6
  Out1 : Outport
  wires:
  Sum4_stage3_pd1/1 -> Out1/1
  Sum4_stage3/1 -> Sum4_stage3_pd1/1
  In2/1 -> Sum4_stage3/2
  In1/1 -> Sum4_stage3/1

== system gm_uz_pmsm_model_6LUT_pd_vnl/uz_pmsm_model/Sum4_stage4 ==
  In1 : Inport
  In2 : Inport  Port=2
  Sum4_stage4 : Sum  Inputs=+-  OutDataTypeStr=single  SampleTime=1e-08
  Sum4_stage4_pd1 : Delay  DelayLength=6
  Out1 : Outport
  wires:
  Sum4_stage4_pd1/1 -> Out1/1
  Sum4_stage4/1 -> Sum4_stage4_pd1/1
  In2/1 -> Sum4_stage4/2
  In1/1 -> Sum4_stage4/1

== system gm_uz_pmsm_model_6LUT_pd_vnl/uz_pmsm_model/Sum5 ==
  In1 : Inport
  In2 : Inport  Port=2
  Sum5 : Sum  Inputs=+-  OutDataTypeStr=single  SampleTime=1e-08
  Sum5_pd1 : Delay  DelayLength=6
  Out1 : Outport
  wires:
  Sum5_pd1/1 -> Out1/1
  Sum5/1 -> Sum5_pd1/1
  In2/1 -> Sum5/2
  In1/1 -> Sum5/1

== system gm_uz_pmsm_model_6LUT_pd_vnl/uz_pmsm_model/Sum51 ==
  In1 : Inport
  In2 : Inport  Port=2
  Sum51 : Sum  OutDataTypeStr=single  SampleTime=1e-08
  Sum51_pd1 : Delay  DelayLength=6
  Out1 : Outport
  wires:
  Sum51_pd1/1 -> Out1/1
  Sum51/1 -> Sum51_pd1/1
  In2/1 -> Sum51/2
  In1/1 -> Sum51/1

== system gm_uz_pmsm_model_6LUT_pd_vnl/uz_pmsm_model/Sum52 ==
  In1 : Inport
  In2 : Inport  Port=2
  Sum52 : Sum  OutDataTypeStr=single  SampleTime=1e-08
  Sum52_pd1 : Delay  DelayLength=6
  Out1 : Outport
  wires:
  Sum52_pd1/1 -> Out1/1
  Sum52/1 -> Sum52_pd1/1
  In2/1 -> Sum52/2
  In1/1 -> Sum52/1

== system gm_uz_pmsm_model_6LUT_pd_vnl/uz_pmsm_model/Sum53 ==
  In1 : Inport
  In2 : Inport  Port=2
  Sum53 : Sum  OutDataTypeStr=single  SampleTime=1e-08
  Sum53_pd1 : Delay  DelayLength=6
  Out1 : Outport
  wires:
  Sum53_pd1/1 -> Out1/1
  Sum53/1 -> Sum53_pd1/1
  In2/1 -> Sum53/2
  In1/1 -> Sum53/1

== system gm_uz_pmsm_model_6LUT_pd_vnl/uz_pmsm_model/Sum6 ==
  In1 : Inport
  In2 : Inport  Port=2
  Sum6 : Sum  Inputs=+-  OutDataTypeStr=single  SampleTime=1e-08
  Sum6_pd1 : Delay  DelayLength=6
  Out1 : Outport
  wires:
  Sum6_pd1/1 -> Out1/1
  Sum6/1 -> Sum6_pd1/1
  In2/1 -> Sum6/2
  In1/1 -> Sum6/1

== system gm_uz_pmsm_model_6LUT_pd_vnl/uz_pmsm_model/Sum7 ==
  In1 : Inport
  In2 : Inport  Port=2
  Sum7 : Sum  Inputs=+-  OutDataTypeStr=single  SampleTime=1e-08
  Sum7_pd1 : Delay  DelayLength=6
  Out1 : Outport
  wires:
  Sum7_pd1/1 -> Out1/1
  Sum7/1 -> Sum7_pd1/1
  In2/1 -> Sum7/2
  In1/1 -> Sum7/1

== system gm_uz_pmsm_model_6LUT_pd_vnl/uz_pmsm_model/Sum71 ==
  In1 : Inport
  In2 : Inport  Port=2
  Sum71 : Sum  Inputs=+-  OutDataTypeStr=single  SampleTime=1e-08
  Sum71_pd1 : Delay  DelayLength=6
  Out1 : Outport
  wires:
  Sum71_pd1/1 -> Out1/1
  Sum71/1 -> Sum71_pd1/1
  In2/1 -> Sum71/2
  In1/1 -> Sum71/1

== system gm_uz_pmsm_model_6LUT_pd_vnl/uz_pmsm_model/Sum8 ==
  In1 : Inport
  In2 : Inport  Port=2
  Sum8 : Sum  Inputs=+-  OutDataTypeStr=single  SampleTime=1e-08
  Sum8_pd1 : Delay  DelayLength=6
  Out1 : Outport
  wires:
  Sum8_pd1/1 -> Out1/1
  Sum8/1 -> Sum8_pd1/1
  In2/1 -> Sum8/2
  In1/1 -> Sum8/1

== system gm_uz_pmsm_model_6LUT_pd_vnl/uz_pmsm_model/Tanh ==
  In1 : Inport
  Tanh : Trigonometry  Operator=tanh  SampleTime=1e-08
  Tanh_pd1 : Delay  DelayLength=25
  Out1 : Outport
  wires:
  Tanh_pd1/1 -> Out1/1
  Tanh/1 -> Tanh_pd1/1
  In1/1 -> Tanh/1

== system gm_uz_pmsm_model_6LUT_pd_vnl/uz_pmsm_model/Tanh1 ==
  In1 : Inport
  Tanh1 : Trigonometry  Operator=cosh  SampleTime=1e-08
  Tanh1_pd1 : Delay  DelayLength=17
  Out1 : Outport
  wires:
  Tanh1_pd1/1 -> Out1/1
  Tanh1/1 -> Tanh1_pd1/1
  In1/1 -> Tanh1/1

== system gm_uz_pmsm_model_6LUT_pd_vnl/uz_pmsm_model/Tanh11 ==
  In1 : Inport
  Tanh11 : Trigonometry  Operator=tanh  SampleTime=1e-08
  Tanh11_pd1 : Delay  DelayLength=25
  Out1 : Outport
  wires:
  Tanh11_pd1/1 -> Out1/1
  Tanh11/1 -> Tanh11_pd1/1
  In1/1 -> Tanh11/1

== system gm_uz_pmsm_model_6LUT_pd_vnl/uz_pmsm_model/Tanh12 ==
  In1 : Inport
  Tanh12 : Trigonometry  Operator=tanh  SampleTime=1e-08
  Tanh12_pd1 : Delay  DelayLength=25
  Out1 : Outport
  wires:
  Tanh12_pd1/1 -> Out1/1
  Tanh12/1 -> Tanh12_pd1/1
  In1/1 -> Tanh12/1

== system gm_uz_pmsm_model_6LUT_pd_vnl/uz_pmsm_model/Tanh13 ==
  In1 : Inport
  Tanh13 : Trigonometry  Operator=cosh  SampleTime=1e-08
  Tanh13_pd1 : Delay  DelayLength=17
  Out1 : Outport
  wires:
  Tanh13_pd1/1 -> Out1/1
  Tanh13/1 -> Tanh13_pd1/1
  In1/1 -> Tanh13/1

== system gm_uz_pmsm_model_6LUT_pd_vnl/uz_pmsm_model/Tanh2 ==
  In1 : Inport
  Tanh2 : Trigonometry  Operator=cosh  SampleTime=1e-08
  Tanh2_pd1 : Delay  DelayLength=17
  Out1 : Outport
  wires:
  Tanh2_pd1/1 -> Out1/1
  Tanh2/1 -> Tanh2_pd1/1
  In1/1 -> Tanh2/1

== system gm_uz_pmsm_model_6LUT_pd_vnl/uz_pmsm_model/Tanh21 ==
  In1 : Inport
  Tanh21 : Trigonometry  Operator=cosh  SampleTime=1e-08
  Tanh21_pd1 : Delay  DelayLength=17
  Out1 : Outport
  wires:
  Tanh21_pd1/1 -> Out1/1
  Tanh21/1 -> Tanh21_pd1/1
  In1/1 -> Tanh21/1

== system gm_uz_pmsm_model_6LUT_pd_vnl/uz_pmsm_model/Tanh3 ==
  In1 : Inport
  Tanh3 : Trigonometry  Operator=cosh  SampleTime=1e-08
  Tanh3_pd1 : Delay  DelayLength=17
  Out1 : Outport
  wires:
  Tanh3_pd1/1 -> Out1/1
  Tanh3/1 -> Tanh3_pd1/1
  In1/1 -> Tanh3/1

== system gm_uz_pmsm_model_6LUT_pd_vnl/uz_pmsm_model/Tanh31 ==
  In1 : Inport
  Tanh31 : Trigonometry  Operator=cosh  SampleTime=1e-08
  Tanh31_pd1 : Delay  DelayLength=17
  Out1 : Outport
  wires:
  Tanh31_pd1/1 -> Out1/1
  Tanh31/1 -> Tanh31_pd1/1
  In1/1 -> Tanh31/1

== system gm_uz_pmsm_model_6LUT_pd_vnl/uz_pmsm_model/Tanh4 ==
  In1 : Inport
  Tanh4 : Trigonometry  Operator=cosh  SampleTime=1e-08
  Tanh4_pd1 : Delay  DelayLength=17
  Out1 : Outport
  wires:
  Tanh4_pd1/1 -> Out1/1
  Tanh4/1 -> Tanh4_pd1/1
  In1/1 -> Tanh4/1

== system gm_uz_pmsm_model_6LUT_pd_vnl/uz_pmsm_model/Tanh41 ==
  In1 : Inport
  Tanh41 : Trigonometry  Operator=cosh  SampleTime=1e-08
  Tanh41_pd1 : Delay  DelayLength=17
  Out1 : Outport
  wires:
  Tanh41_pd1/1 -> Out1/1
  Tanh41/1 -> Tanh41_pd1/1
  In1/1 -> Tanh41/1

== system gm_uz_pmsm_model_6LUT_pd_vnl/uz_pmsm_model/Tanh5 ==
  In1 : Inport
  Tanh5 : Trigonometry  Operator=tanh  SampleTime=1e-08
  Tanh5_pd1 : Delay  DelayLength=25
  Out1 : Outport
  wires:
  Tanh5_pd1/1 -> Out1/1
  Tanh5/1 -> Tanh5_pd1/1
  In1/1 -> Tanh5/1

== system gm_uz_pmsm_model_6LUT_pd_vnl/uz_pmsm_model_vnl/mechanical_system ==
  note: This delay breaks the algebraic loop between mechanical and electrical system.
      | Introduces a delay of 500ns.
  reset : Inport
  M_Mi : Inport  Port=2
  mu : Inport  Port=3
  M_n0 : Inport  Port=4
  reciprocal_J : Inport  Port=5
  load_torque : Inport  Port=6
  Abs : Abs  SaturateOnIntegerOverflow=off
  Delay : Delay  DelayLength=1
  Product11 : Product
  Product12 : Product
  Product4 : Product
  Sign1 : Signum
  Sum : Sum  Inputs=|+-
  Sum1 : Sum  Inputs=|+-
  Sum5 : Sum  Inputs=|++
  integrator1 : Subsystem
  omega_mech : Outport
  wires:
  Delay/1 -> Sum1/1
  Product4/1 -> Sum/2
  Sum/1 -> Delay/1
  load_torque/1 -> Sum1/2
  Sum1/1 -> Product11/2
  M_Mi/1 -> Sum/1
  reciprocal_J/1 -> Product11/1
  M_n0/1 -> Sum5/2
  mu/1 -> Product12/1
  Product12/1 -> Sum5/1
  reset/1 -> integrator1/1(reset)
  Abs/1 -> Product12/2
  integrator1/1(outt) -> omega_mech/1, Abs/1, Sign1/1
  Sign1/1 -> Product4/2
  Sum5/1 -> Product4/1
  Product11/1 -> integrator1/2(in)

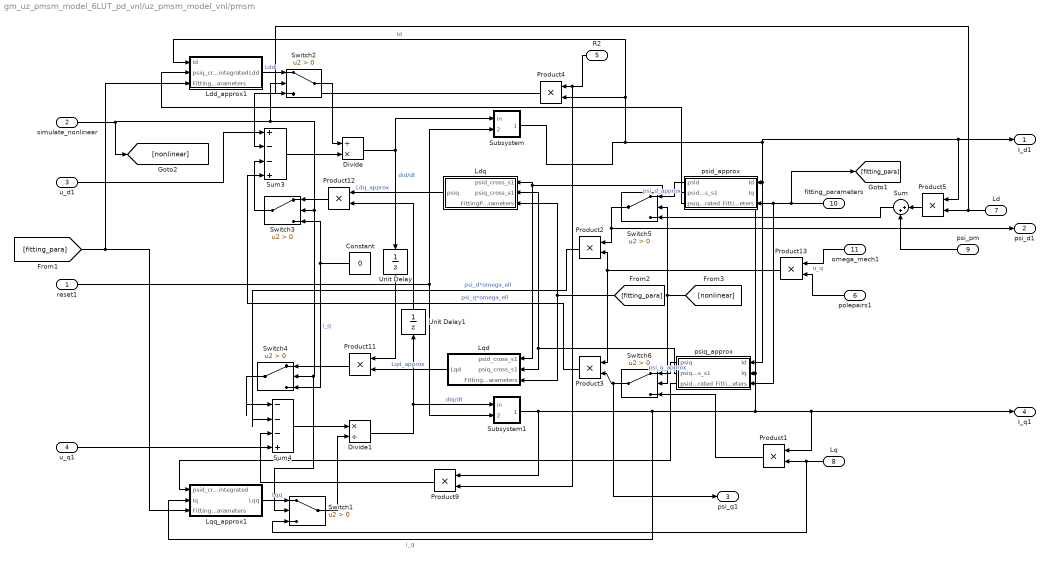
== system gm_uz_pmsm_model_6LUT_pd_vnl/uz_pmsm_model_vnl/pmsm ==
  reset1 : Inport
  simulate_nonlinear : Inport  Port=2
  u_d1 : Inport  Port=3
  u_q1 : Inport  Port=4
  R2 : Inport  Port=5
  polepairs1 : Inport  Port=6
  Ld : Inport  Port=7
  Lq : Inport  Port=8
  psi_pm : Inport  Port=9
  fitting_parameters : Inport  Port=10
  omega_mech1 : Inport  Port=11
  Constant : Constant  Value=0  OutDataTypeStr=single  SampleTime=ts
  Divide : Product  Inputs=/*  OutDataTypeStr=Inherit: Same as first input
  Divide1 : Product  Inputs=*/  OutDataTypeStr=Inherit: Same as first input
  Ldd_approx1 : Subsystem
  Ldq : Subsystem
  Lqd : Subsystem
  Lqq_approx1 : Subsystem
  Product1 : Product
  Product11 : Product
  Product{2,4..5,9,12..13} (6 alike) : Product  OutDataTypeStr=Inherit: Same as first input
  Product3 : Product
  Subsystem : Subsystem
  Subsystem1 : Subsystem
  Sum : Sum  Inputs=|++  OutDataTypeStr=Inherit: Same as first input
  Sum3 : Sum  Inputs=|+--+  OutDataTypeStr=Inherit: Same as first input
  Sum4 : Sum  Inputs=|---+
  Switch{1..6} (6 alike) : Switch  Criteria=u2 > Threshold  SaturateOnIntegerOverflow=off  InputSameDT=off
  Unit Delay : UnitDelay  SampleTime=-1  HasFrameUpgradeWarning=on
  Unit Delay1 : UnitDelay  SampleTime=-1  HasFrameUpgradeWarning=on
  psid_approx : Subsystem
  psiq_approx : Subsystem
  I_d1 : Outport
  psi_d1 : Outport  Port=2
  psi_q1 : Outport  Port=3
  I_q1 : Outport  Port=4
  wires:
  Constant/1 -> Switch3/3, Switch4/3  "i_q"
  psid_approx/3(psiq_cross_s1_integrated) -> Ldd_approx1/2(psiq_cross_s1_integrated)
  psiq_approx/3(psid_cross_s1_integrated) -> Lqq_approx1/1(psid_cross_s1_integrated)
  psid_approx/2(psid_cross_s1) -> Lqd/1(psid_cross_s1), Ldq/1(psid_cross_s1)
  psiq_approx/2(psiq_cross_s1) -> Ldq/2(psiq_cross_s1), Lqd/2(psiq_cross_s1)
  [fitting_para] -> Lqd/3(FittingParameters), Ldq/3(FittingParameters)
  [fitting_para] -> Lqq_approx1/3(FittingParameters), Ldd_approx1/3(FittingParameters)
  Product1/1 -> Switch6/3
  Lq/1 -> Product1/2, Switch1/3
  [nonlinear] -> Switch6/2, Switch5/2
  Switch6/1 -> Product3/2, psi_q1/1
  psiq_approx/1(psiq) -> Switch6/1  "psi_q_approx"
  Sum/1 -> Switch5/3
  psi_pm/1 -> Sum/2
  Ld/1 -> Product5/2, Switch2/3
  Product5/1 -> Sum/1
  Switch5/1 -> Product2/1, psi_d1/1
  psid_approx/1(psid) -> Switch5/1  "psi_d_approx"
  simulate_nonlinear/1 -> [nonlinear], Switch2/2, Switch3/2, Switch4/2, Switch1/2
  Switch4/1 -> Sum4/1
  Product11/1 -> Switch4/1
  Switch3/1 -> Sum3/3
  Product12/1 -> Switch3/1
  Switch2/1 -> Divide/1
  Ldd_approx1/1(Ldd) -> Switch2/1  "Ldd"
  Switch1/1 -> Divide1/2
  Lqq_approx1/1(Lqq) -> Switch1/1  "Lqq"
  fitting_parameters/1 -> psid_approx/3(FittingParameters), psiq_approx/3(FittingParameters), [fitting_para]
  omega_mech1/1 -> Product13/1  "u_q"
  Ldq/1(psiq) -> Product12/1  "Ldq_approx"
  Lqd/1(Lqd) -> Product11/2  "Lqd_approx"
  Unit Delay1/1 -> Product12/2
  Unit Delay/1 -> Product11/1
  Product2/1 -> Sum4/2  "psi_d*omega_ell"
  Product4/1 -> Sum3/2
  Product3/1 -> Sum3/4  "psi_q*omega_ell"
  Subsystem1/1(outt) -> Product9/1, psiq_approx/2(Iq), psid_approx/2(Iq), Product1/1, I_q1/1, Lqq_approx1/2(Iq)  "i_q"
  Subsystem/1(outt) -> psiq_approx/1(Id), psid_approx/1(Id), I_d1/1, Product5/1, Product4/2, Ldd_approx1/1(Id)  "id"
  R2/1 -> Product4/1, Product9/2
  u_d1/1 -> Sum3/1
  reset1/1 -> Subsystem1/2(reset), Subsystem/2(reset)
  Product9/1 -> Sum4/3
  Sum3/1 -> Divide/2
  Divide/1 -> Subsystem/1(in), Unit Delay/1  "did/dt"
  Product13/1 -> Product2/2, Product3/1
  polepairs1/1 -> Product13/2
  Divide1/1 -> Subsystem1/1(in), Unit Delay1/1  "diq/dt"
  u_q1/1 -> Sum4/4
  Sum4/1 -> Divide1/1

== system gm_uz_pmsm_model_6LUT_pd_vnl/uz_pmsm_model_vnl/torque_calculation ==
  I_d : Inport
  psi_d : Inport  Port=2
  psi_q : Inport  Port=3
  polepairs : Inport  Port=4
  I_q : Inport  Port=5
  Factor : Gain  Gain=(3/2)
  Product2 : Product
  Product3 : Product
  Product9 : Product
  Sum3 : Sum  Inputs=-|+
  M_Mi : Outport
  wires:
  Factor/1 -> Product9/1  "M_Mi"
  polepairs/1 -> Product9/2
  Product9/1 -> M_Mi/1  "M_Mi"
  I_q/1 -> Product3/2
  I_d/1 -> Product2/1
  psi_d/1 -> Product3/1
  psi_q/1 -> Product2/2
  Product2/1 -> Sum3/1
  Product3/1 -> Sum3/2
  Sum3/1 -> Factor/1

== system gm_uz_pmsm_model_6LUT_pd_vnl/Compare/Assert_outputs/RelErrCheck ==
  In1 : Inport
  In2 : Inport  Port=2
  "RelativeErrorCheck " : MATLAB Function  TreatAsAtomicUnit=on
  Out1 : Outport  VectorParamsAs1DForOutWhenUnconnected=off
  wires:
  "RelativeErrorCheck "/1(y) -> Out1/1
  In1/1 -> "RelativeErrorCheck "/1(P)
  In2/1 -> "RelativeErrorCheck "/2(R)

== system gm_uz_pmsm_model_6LUT_pd_vnl/Current_Controller/Entkopplungen/Lineare_Entkopplung ==
  i_d : Inport
  i_q : Inport  Port=2
  omega_m : Inport  Port=3
  Constant1 : Constant  Value=psi_pm  SampleTime=-1
  Gain : Gain  Gain=L_q
  Gain1 : Gain  Gain=L_d
  Gain2 : Gain  Gain=polepair
  Product : Product
  Product1 : Product
  Sum6 : Sum  Inputs=|++
  u_d : Outport
  u_q : Outport  Port=2
  wires:
  omega_m/1 -> Gain2/1
  Sum6/1 -> Product1/1
  Product/1 -> u_d/1
  i_d/1 -> Gain1/1
  Constant1/1 -> Sum6/2
  i_q/1 -> Gain/1
  Product1/1 -> u_q/1
  Gain1/1 -> Sum6/1
  Gain2/1 -> Product1/2, Product/2
  Gain/1 -> Product/1

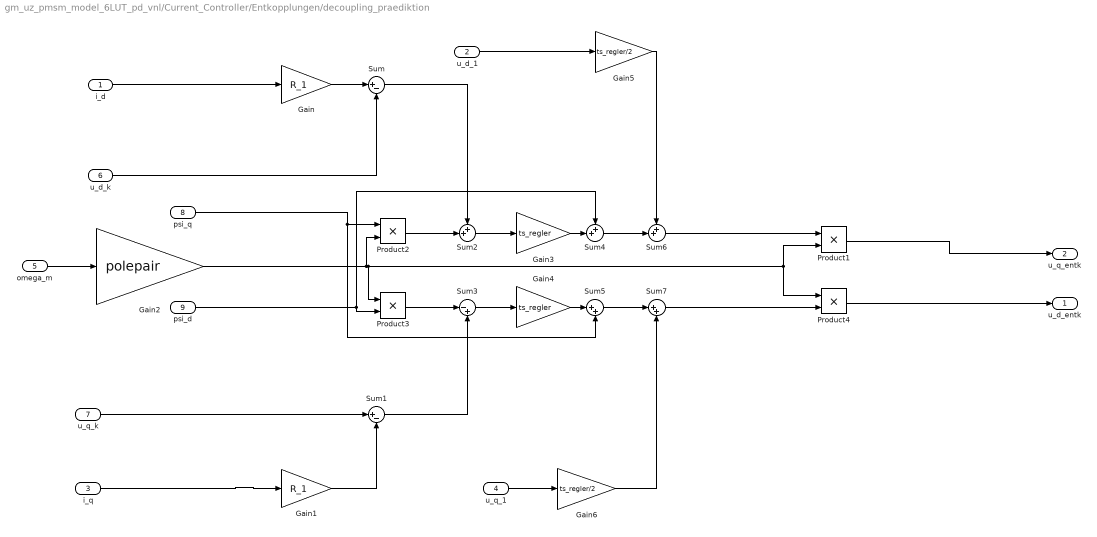
== system gm_uz_pmsm_model_6LUT_pd_vnl/Current_Controller/Entkopplungen/decoupling_praediktion ==
  i_d : Inport
  u_d_1 : Inport  Port=2
  i_q : Inport  Port=3
  u_q_1 : Inport  Port=4
  omega_m : Inport  Port=5
  u_d_k : Inport  Port=6
  u_q_k : Inport  Port=7
  psi_q : Inport  Port=8
  psi_d : Inport  Port=9
  Gain : Gain  Gain=R_1
  Gain1 : Gain  Gain=R_1
  Gain2 : Gain  Gain=polepair
  Gain3 : Gain  Gain=ts_regler
  Gain4 : Gain  Gain=ts_regler
  Gain5 : Gain  Gain=ts_regler/2
  Gain6 : Gain  Gain=ts_regler/2
  Product{1..4} (4 alike) : Product
  Sum : Sum  Inputs=|+-
  Sum1 : Sum  Inputs=|+-
  Sum2 : Sum  Inputs=++|
  Sum3 : Sum  Inputs=|-+
  Sum4 : Sum  Inputs=++|
  Sum5 : Sum  Inputs=|++
  Sum6 : Sum  Inputs=++|
  Sum7 : Sum  Inputs=|++
  u_d_entk : Outport
  u_q_entk : Outport  Port=2
  wires:
  psi_q/1 -> Sum5/2, Product2/1
  psi_d/1 -> Product3/2, Sum4/1
  Gain2/1 -> Product1/2, Product4/1, Product3/1, Product2/2
  u_d_k/1 -> Sum/2
  Gain/1 -> Sum/1
  u_q_k/1 -> Sum1/1
  Gain1/1 -> Sum1/2
  Product3/1 -> Sum3/1
  Product2/1 -> Sum2/2
  Sum/1 -> Sum2/1
  Sum1/1 -> Sum3/2
  Sum3/1 -> Gain4/1
  Sum2/1 -> Gain3/1
  Gain3/1 -> Sum4/2
  Gain4/1 -> Sum5/1
  u_d_1/1 -> Gain5/1
  Sum4/1 -> Sum6/2
  u_q_1/1 -> Gain6/1
  Gain5/1 -> Sum6/1
  Sum5/1 -> Sum7/1
  Gain6/1 -> Sum7/2
  Sum6/1 -> Product1/1
  Sum7/1 -> Product4/2
  omega_m/1 -> Gain2/1
  i_d/1 -> Gain/1
  i_q/1 -> Gain1/1
  Product1/1 -> u_q_entk/1
  Product4/1 -> u_d_entk/1

== system gm_uz_pmsm_model_6LUT_pd_vnl/Current_Controller/Entkopplungen/dynamic_nonlinear_entkopplung1 ==
  i_d : Inport
  i_q : Inport  Port=2
  psi_d : Inport  Port=3
  psi_q : Inport  Port=4
  Ldq_LUT : Inport  Port=5
  Lqd_LUT : Inport  Port=6
  omega_m : Inport  Port=7
  Gain2 : Gain  Gain=polepair
  Product{,1..3} (4 alike) : Product
  Sum1 : Sum  Inputs=++|
  Sum6 : Sum  Inputs=++|
  u_d : Outport
  u_q : Outport  Port=2
  wires:
  psi_q/1 -> Product/1  "psi_q_LUT"
  Gain2/1 -> Product1/2, Product/2
  psi_d/1 -> Product1/1  "psi_d_LUT"
  omega_m/1 -> Gain2/1
  i_d/1 -> Product2/1
  Ldq_LUT/1 -> Product2/2
  Sum6/1 -> u_q/1
  Product1/1 -> Sum6/2
  Product/1 -> Sum1/2
  Sum1/1 -> u_d/1
  i_q/1 -> Product3/1
  Lqd_LUT/1 -> Product3/2
  Product3/1 -> Sum6/1
  Product2/1 -> Sum1/1

== system gm_uz_pmsm_model_6LUT_pd_vnl/Current_Controller/Entkopplungen/static_nonlinear_entkopplung ==
  psi_d : Inport
  psi_q : Inport  Port=2
  omega_m : Inport  Port=3
  Gain2 : Gain  Gain=polepair
  Product : Product
  Product1 : Product
  Scope : Scope  NumInputPorts=2
  u_d : Outport
  u_q : Outport  Port=2
  wires:
  psi_q/1 -> Product/1  "psi_q_LUT"
  Gain2/1 -> Product1/2, Product/2
  Product1/1 -> Scope/1, u_q/1
  Product/1 -> Scope/2, u_d/1
  psi_d/1 -> Product1/1  "psi_d_LUT"
  omega_m/1 -> Gain2/1

== system gm_uz_pmsm_model_6LUT_pd_vnl/uz_pmsm_model_vnl/mechanical_system/integrator1 ==
  reset : Inport
  in : Inport  Port=2
  Delay1 : Delay  DelayLength=1  ExternalReset=Level
      settings: InputPortMap=u0,r5
  Gain : Gain  Gain=ts
  Sum3 : Sum  Inputs=|++
  outt : Outport
  wires:
  Delay1/1 -> outt/1, Sum3/2
  Sum3/1 -> Delay1/1
  reset/1 -> Delay1/2
  Gain/1 -> Sum3/1
  in/1 -> Gain/1

== system gm_uz_pmsm_model_6LUT_pd_vnl/uz_pmsm_model_vnl/pmsm/Ldd_approx1 ==
  Id : Inport
  psiq_cross_s1_integrated : Inport  Port=2
  FittingParameters : Inport  Port=3
  Demux : Demux  Outputs=23
  Product{,1..3} (4 alike) : Product  OutDataTypeStr=single
  Product10 : Product  Inputs=3  OutDataTypeStr=single
  Product14 : Product
  Product15 : Product
  Reciprocal : Product  Inputs=/  RndMeth=Zero  SaturateOnIntegerOverflow=on
  Reciprocal1 : Product  Inputs=/  RndMeth=Zero  SaturateOnIntegerOverflow=on
  Sum : Sum  Inputs=|+-  OutDataTypeStr=single
  Sum1 : Sum  Inputs=|+-  OutDataTypeStr=single
  Sum2 : Sum  Inputs=|+-
  Sum7 : Sum  Inputs=|+-
  Tanh1 : Trigonometry  Operator=cosh
  Tanh4 : Trigonometry  Operator=cosh
  Ldd : Outport
  wires:
  Demux/16 -> Product1/2  "ad1*ad2"
  Demux/15 -> Product3/2  "ad4*ad5"
  Reciprocal/1 -> Product1/1
  psiq_cross_s1_integrated/1 -> Product10/2
  Product2/1 -> Tanh1/1
  Product/1 -> Tanh4/1
  Product14/1 -> Reciprocal/1
  Product15/1 -> Reciprocal1/1
  Reciprocal1/1 -> Product3/1
  Tanh1/1 -> Product15/1, Product15/2
  Tanh4/1 -> Product14/2, Product14/1
  Demux/13 -> Product10/3  "F1G1"
  Sum7/1 -> Ldd/1  "psid_cross_s1"
  Product10/1 -> Sum7/2  "psid_cross"
  Sum2/1 -> Product10/1  "psid_cross_s1_abgeleitet"
  Product3/1 -> Sum2/2  "psid_s1"
  Id/1 -> Sum/1, Sum1/1
  Demux/6 -> Sum1/2  "ad6"
  Demux/5 -> Product2/2  "ad5"
  Sum1/1 -> Product2/1
  Product1/1 -> Sum2/1, Sum7/1  "psidself_abgeleitet"
  Demux/2 -> Product/2  "ad2"
  Sum/1 -> Product/1
  Demux/3 -> Sum/2  "ad3"
  FittingParameters/1 -> Demux/1

== system gm_uz_pmsm_model_6LUT_pd_vnl/uz_pmsm_model_vnl/pmsm/Ldq ==
  psid_cross_s1 : Inport
  psiq_cross_s1 : Inport  Port=2
  FittingParameters : Inport  Port=3
  Gain : Gain  Gain=-1
  Product20 : Product  Inputs=3
  Selector : Selector  InputPortWidth=23  IndexOptions=Index vector (dialog)  Indices=[13]  OutputSizes=1
  psiq : Outport
  wires:
  Selector/1 -> Product20/3
  FittingParameters/1 -> Selector/1
  psiq_cross_s1/1 -> Product20/2
  Gain/1 -> psiq/1
  psid_cross_s1/1 -> Product20/1
  Product20/1 -> Gain/1  "psiq_cross"

== system gm_uz_pmsm_model_6LUT_pd_vnl/uz_pmsm_model_vnl/pmsm/Lqd ==
  psid_cross_s1 : Inport
  psiq_cross_s1 : Inport  Port=2
  FittingParameters : Inport  Port=3
  Gain : Gain  Gain=-1
  Product20 : Product  Inputs=3
  Selector : Selector  InputPortWidth=23  IndexOptions=Index vector (dialog)  Indices=[14]  OutputSizes=1
  Lqd : Outport
  wires:
  Selector/1 -> Product20/3
  psiq_cross_s1/1 -> Product20/2
  Gain/1 -> Lqd/1
  psid_cross_s1/1 -> Product20/1
  Product20/1 -> Gain/1
  FittingParameters/1 -> Selector/1

== system gm_uz_pmsm_model_6LUT_pd_vnl/uz_pmsm_model_vnl/pmsm/Lqq_approx1 ==
  psid_cross_s1_integrated : Inport
  Iq : Inport  Port=2
  FittingParameters : Inport  Port=3
  Demux : Demux  Outputs=23
  Product : Product  OutDataTypeStr=Inherit: Same as first input
  Product{1,3,14..15} (4 alike) : Product
  Product2 : Product  OutDataTypeStr=Inherit: Same as first input
  Product20 : Product  Inputs=3
  Reciprocal : Product  Inputs=/  RndMeth=Zero  SaturateOnIntegerOverflow=on
  Reciprocal1 : Product  Inputs=/  RndMeth=Zero  SaturateOnIntegerOverflow=on
  Sum1 : Sum  Inputs=|++
  Sum10 : Sum  Inputs=|+-
  Sum2 : Sum  Inputs=|+-
  Sum4 : Sum  Inputs=|++
  Tanh1 : Trigonometry  Operator=cosh
  Tanh3 : Trigonometry  Operator=cosh
  Lqq : Outport
  wires:
  Demux/17 -> Product3/2  "aq4*aq5"
  Demux/18 -> Product1/2  "aq1*aq2"
  psid_cross_s1_integrated/1 -> Product20/2
  Product14/1 -> Reciprocal/1
  Product/1 -> Tanh3/1
  Product2/1 -> Tanh1/1
  Product15/1 -> Reciprocal1/1
  Product3/1 -> Sum4/1  "psid_s1"
  Sum4/1 -> Sum2/2
  Sum1/1 -> Sum2/1, Sum10/1
  Product1/1 -> Sum1/1  "psidself_abgeleitet"
  Demux/11 -> Product2/2  "aq5"
  Iq/1 -> Product/1, Product2/1
  Demux/8 -> Product/2  "aq2"
  Reciprocal1/1 -> Product3/1
  Reciprocal/1 -> Product1/1
  Sum2/1 -> Product20/1
  Tanh1/1 -> Product15/1, Product15/2
  Tanh3/1 -> Product14/2, Product14/1
  Demux/9 -> Sum1/2  "aq3"
  Demux/14 -> Product20/3
  Sum10/1 -> Lqq/1  "Lqq"
  Product20/1 -> Sum10/2  "psiq_cross"
  Demux/12 -> Sum4/2  "aq6"
  FittingParameters/1 -> Demux/1

== system gm_uz_pmsm_model_6LUT_pd_vnl/uz_pmsm_model_vnl/pmsm/Subsystem ==
  in : Inport
  reset : Inport  Port=2
  Delay1 : Delay  DelayLength=1  ExternalReset=Level
      settings: InputPortMap=u0,r5
  Gain7 : Gain  Gain=ts
  Sum5 : Sum  Inputs=|++
  outt : Outport
  wires:
  Gain7/1 -> Sum5/1  "u_d"
  Sum5/1 -> Delay1/1
  Delay1/1 -> Sum5/2, outt/1
  reset/1 -> Delay1/2
  in/1 -> Gain7/1

== system gm_uz_pmsm_model_6LUT_pd_vnl/uz_pmsm_model_vnl/pmsm/Subsystem1 ==
  in : Inport
  reset : Inport  Port=2
  Delay1 : Delay  DelayLength=1  ExternalReset=Level
      settings: InputPortMap=u0,r5
  Gain7 : Gain  Gain=ts
  Sum5 : Sum  Inputs=|++
  outt : Outport
  wires:
  Gain7/1 -> Sum5/1  "u_d"
  Sum5/1 -> Delay1/1
  Delay1/1 -> Sum5/2, outt/1
  reset/1 -> Delay1/2
  in/1 -> Gain7/1
